simulink model "Both_Systems_GUI"  (R2020b)
settings: Solver=VariableStepAuto  StartTime=0.0  StopTime=10.0  RelTol=1e-3
model workspace (MAT data in the model file):
  Elev_Anti_friction = Simulink.Parameter
  Elev_Anti_friction.Value = 1
  Elev_Anti_friction.DataType = 'auto'
  Elev_Anti_friction.Dimensions = [1 1]
  Elev_Backlash = Simulink.Parameter
  Elev_Backlash.Value = 1
  Elev_Backlash.DataType = 'auto'
  Elev_Backlash.Dimensions = [1 1]
  Elev_CL = Simulink.Parameter
  Elev_CL.Value = 1
  Elev_CL.DataType = 'auto'
  Elev_CL.Dimensions = [1 1]
  Elev_Dist = Simulink.Parameter
  Elev_Dist.Value = 0
  Elev_Dist.DataType = 'auto'
  Elev_Dist.Dimensions = [1 1]
  Elev_Gun_Step = Simulink.Parameter
  Elev_Gun_Step.Value = 0
  Elev_Gun_Step.DataType = 'auto'
  Elev_Gun_Step.Dimensions = [1 1]
  Elev_Gun_Step_1_or_0_05 = Simulink.Parameter
  Elev_Gun_Step_1_or_0_05.Value = 1
  Elev_Gun_Step_1_or_0_05.DataType = 'auto'
  Elev_Gun_Step_1_or_0_05.Dimensions = [1 1]
  Elev_Input = Simulink.Parameter
  Elev_Input.Value = 1
  Elev_Input.DataType = 'auto'
  Elev_Input.Dimensions = [1 1]
  Elev_Insert_Input = Simulink.Parameter
  Elev_Insert_Input.Value = 0
  Elev_Insert_Input.DataType = 'auto'
  Elev_Insert_Input.Dimensions = [1 1]
  Elev_Optics_Enabled = Simulink.Parameter
  Elev_Optics_Enabled.Value = 1
  Elev_Optics_Enabled.DataType = 'auto'
  Elev_Optics_Enabled.Dimensions = [1 1]
  Elev_Pod_Backlash = Simulink.Parameter
  Elev_Pod_Backlash.Value = 1
  Elev_Pod_Backlash.DataType = 'auto'
  Elev_Pod_Backlash.Dimensions = [1 1]
  Elev_Pod_CL = Simulink.Parameter
  Elev_Pod_CL.Value = 1
  Elev_Pod_CL.DataType = 'auto'
  Elev_Pod_CL.Dimensions = [1 1]
  Elev_Pod_Friction = Simulink.Parameter
  Elev_Pod_Friction.Value = 1
  Elev_Pod_Friction.DataType = 'auto'
  Elev_Pod_Friction.Dimensions = [1 1]
  Elev_Pod_Step = Simulink.Parameter
  Elev_Pod_Step.Value = 0
  Elev_Pod_Step.DataType = 'auto'
  Elev_Pod_Step.Dimensions = [1 1]
  Elev_Pod_Step_1_or_0_05 = Simulink.Parameter
  Elev_Pod_Step_1_or_0_05.Value = 1
  Elev_Pod_Step_1_or_0_05.DataType = 'auto'
  Elev_Pod_Step_1_or_0_05.Dimensions = [1 1]
  Elev_Pod_Tacho = Simulink.Parameter
  Elev_Pod_Tacho.Value = 0
  Elev_Pod_Tacho.DataType = 'auto'
  Elev_Pod_Tacho.Dimensions = [1 1]
  Elev_Pod_hold = Simulink.Parameter
  Elev_Pod_hold.Value = 1
  Elev_Pod_hold.DataType = 'auto'
  Elev_Pod_hold.Dimensions = [1 1]
  Elev_Step_1_or_0_05 = Simulink.Parameter
  Elev_Step_1_or_0_05.Value = 1
  Elev_Step_1_or_0_05.DataType = 'auto'
  Elev_Step_1_or_0_05.Dimensions = [1 1]
  Elev_Tacho = Simulink.Parameter
  Elev_Tacho.Value = 0
  Elev_Tacho.DataType = 'auto'
  Elev_Tacho.Dimensions = [1 1]
  Elev_diffrentiator = Simulink.Parameter
  Elev_diffrentiator.Value = 1
  Elev_diffrentiator.DataType = 'auto'
  Elev_diffrentiator.Dimensions = [1 1]
  Elev_fire = Simulink.Parameter
  Elev_fire.Value = 1
  Elev_fire.DataType = 'auto'
  Elev_fire.Dimensions = [1 1]
  Elev_friction = Simulink.Parameter
  Elev_friction.Value = 1
  Elev_friction.DataType = 'auto'
  Elev_friction.Dimensions = [1 1]
  Trav_Anti_friction = Simulink.Parameter
  Trav_Anti_friction.Value = 1
  Trav_Anti_friction.DataType = 'auto'
  Trav_Anti_friction.Dimensions = [1 1]
  Trav_Backlash = Simulink.Parameter
  Trav_Backlash.Value = 1
  Trav_Backlash.DataType = 'auto'
  Trav_Backlash.Dimensions = [1 1]
  Trav_CL = Simulink.Parameter
  Trav_CL.Value = 1
  Trav_CL.DataType = 'auto'
  Trav_CL.Dimensions = [1 1]
  Trav_Dist = Simulink.Parameter
  Trav_Dist.Value = 1
  Trav_Dist.DataType = 'auto'
  Trav_Dist.Dimensions = [1 1]
  Trav_Gun_Step = Simulink.Parameter
  Trav_Gun_Step.Value = 0
  Trav_Gun_Step.DataType = 'auto'
  Trav_Gun_Step.Dimensions = [1 1]
  Trav_Gun_Step_1_or_0_05 = Simulink.Parameter
  Trav_Gun_Step_1_or_0_05.Value = 1
  Trav_Gun_Step_1_or_0_05.DataType = 'auto'
  Trav_Gun_Step_1_or_0_05.Dimensions = [1 1]
  Trav_Input = Simulink.Parameter
  Trav_Input.Value = 1
  Trav_Input.DataType = 'auto'
  Trav_Input.Dimensions = [1 1]
  Trav_Insert_Input = Simulink.Parameter
  Trav_Insert_Input.Value = 1
  Trav_Insert_Input.DataType = 'auto'
  Trav_Insert_Input.Dimensions = [1 1]
  Trav_Optics_Enabled = Simulink.Parameter
  Trav_Optics_Enabled.Value = 1
  Trav_Optics_Enabled.DataType = 'auto'
  Trav_Optics_Enabled.Dimensions = [1 1]
  Trav_Pod_Backlash = Simulink.Parameter
  Trav_Pod_Backlash.Value = 1
  Trav_Pod_Backlash.DataType = 'auto'
  Trav_Pod_Backlash.Dimensions = [1 1]
  Trav_Pod_CL = Simulink.Parameter
  Trav_Pod_CL.Value = 1
  Trav_Pod_CL.DataType = 'auto'
  Trav_Pod_CL.Dimensions = [1 1]
  Trav_Pod_Friction = Simulink.Parameter
  Trav_Pod_Friction.Value = 1
  Trav_Pod_Friction.DataType = 'auto'
  Trav_Pod_Friction.Dimensions = [1 1]
  Trav_Pod_Step = Simulink.Parameter
  Trav_Pod_Step.Value = 0
  Trav_Pod_Step.DataType = 'auto'
  Trav_Pod_Step.Dimensions = [1 1]
  Trav_Pod_Step_1_or_0_05 = Simulink.Parameter
  Trav_Pod_Step_1_or_0_05.Value = 1
  Trav_Pod_Step_1_or_0_05.DataType = 'auto'
  Trav_Pod_Step_1_or_0_05.Dimensions = [1 1]
  Trav_Pod_Tacho = Simulink.Parameter
  Trav_Pod_Tacho.Value = 0
  Trav_Pod_Tacho.DataType = 'auto'
  Trav_Pod_Tacho.Dimensions = [1 1]
  Trav_Pod_hold = Simulink.Parameter
  Trav_Pod_hold.Value = 1
  Trav_Pod_hold.DataType = 'auto'
  Trav_Pod_hold.Dimensions = [1 1]
  Trav_Step_1_or_0_05 = Simulink.Parameter
  Trav_Step_1_or_0_05.Value = 1
  Trav_Step_1_or_0_05.DataType = 'auto'
  Trav_Step_1_or_0_05.Dimensions = [1 1]
  Trav_Tacho = Simulink.Parameter
  Trav_Tacho.Value = 0
  Trav_Tacho.DataType = 'auto'
  Trav_Tacho.Dimensions = [1 1]
  Trav_diffrentiator = Simulink.Parameter
  Trav_diffrentiator.Value = 1
  Trav_diffrentiator.DataType = 'auto'
  Trav_diffrentiator.Dimensions = [1 1]
  Trav_fire = Simulink.Parameter
  Trav_fire.Value = 1
  Trav_fire.DataType = 'auto'
  Trav_fire.Dimensions = [1 1]
  Trav_friction = Simulink.Parameter
  Trav_friction.Value = 1
  Trav_friction.DataType = 'auto'
  Trav_friction.Dimensions = [1 1]
libraries: simulink x1
settings Model: Creator=דניאל ואיתי  LastModifiedBy=דניאל ואיתי

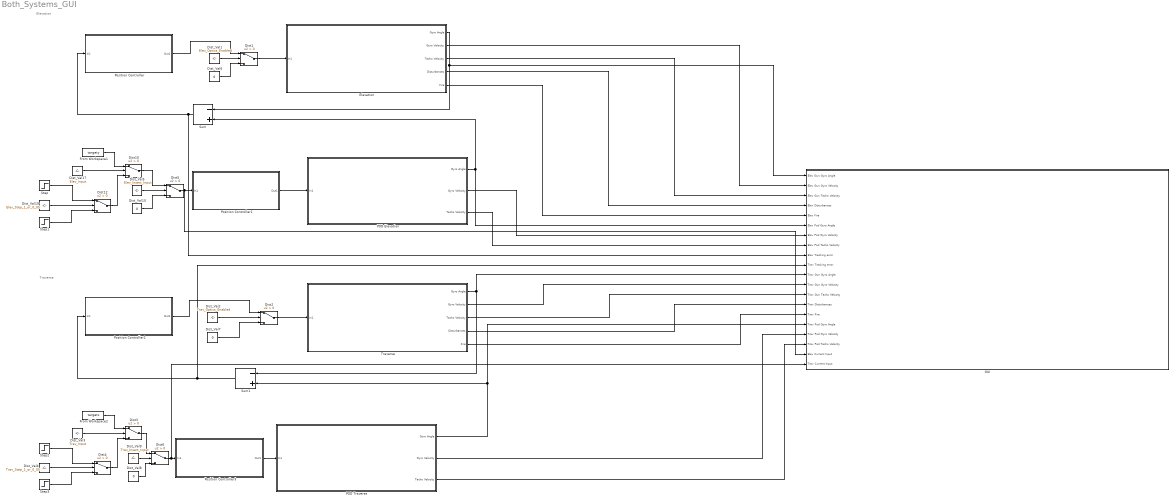
== system Both_Systems_GUI ==
  note: Elevation
  note: Traverse
  Dist{1..6,10,12} (8 alike) : Switch  Criteria=u2 > Threshold
  Dist_Val1 : Constant  Value=Elev_Optics_Enabled
  Dist_Val{6..8,10} (4 alike) : Constant  Value=0
  Dist_Val17 : Constant  Value=Elev_Input
  Dist_Val19 : Constant  Value=Elev_Step_1_or_0_05  VectorParams1D=off
  Dist_Val2 : Constant  Value=Trav_Optics_Enabled
  Dist_Val3 : Constant  Value=Trav_Input
  Dist_Val4 : Constant  Value=Trav_Step_1_or_0_05  VectorParams1D=off
  Dist_Val5 : Constant  Value=Elev_Insert_Input
  Dist_Val9 : Constant  Value=Trav_Insert_Input
  Elevation : Subsystem
  From Workspace1 : FromWorkspace  VariableName=targety
  From Workspace2 : FromWorkspace  VariableName=targetx
  GUI : Subsystem
  POD Elevation : Subsystem
  POD Traverse : Subsystem
  Position Controller : Subsystem
  Position Controller1 : Subsystem
  Position Controller2 : Subsystem
  Position Controller3 : Subsystem
  Step : Step  SampleTime=0
  Step1 : Step  After=0.05  SampleTime=0
  Step2 : Step  SampleTime=0
  Step3 : Step  After=0.05  SampleTime=0
  Sum : Sum  Inputs=-+
  Sum1 : Sum  Inputs=-+
  Traverse : Subsystem
  wires:
  Position Controller1/1(Out1) -> POD Elevation/1(In1)
  POD Elevation/2(Gyro Velocity) -> GUI/7(Elev Pod Gyro Velocity)
  Dist_Val17/1 -> Dist10/2
  From Workspace1/1 -> Dist10/1
  Step1/1 -> Dist12/3
  Elevation/3(Tacho Velocity) -> GUI/3(Elev Gun Tacho Velocity)
  POD Elevation/3(Tacho Velocity) -> GUI/8(Elev Pod Tacho Velocity)
  Elevation/2(Gyro Velocity) -> GUI/2(Elev Gun Gyro Velocity)
  Dist_Val1/1 -> Dist1/2
  Elevation/4(Disturbances) -> GUI/4(Elev Disturbances)
  POD Elevation/1(Gyro Angle) -> Sum/2, GUI/6(Elev Pod Gyro Angle)
  Step/1 -> Dist12/1
  Dist_Val19/1 -> Dist12/2
  Elevation/5(Fire) -> GUI/5(Elev Fire)
  Dist1/1 -> Elevation/1(In1)
  Dist12/1 -> Dist10/3
  Position Controller/1(Out1) -> Dist1/1
  Elevation/1(Gyro Angle) -> GUI/1(Elev Gun Gyro Angle), Sum/1
  Position Controller3/1(Out1) -> POD Traverse/1(In1)
  Dist2/1 -> Traverse/1(In1)
  Step2/1 -> Dist4/1
  Sum1/1 -> Position Controller2/1(In1), GUI/10(Trav Tracking error)
  From Workspace2/1 -> Dist3/1
  Dist4/1 -> Dist3/3
  Position Controller2/1(Out1) -> Dist2/1
  Step3/1 -> Dist4/3
  Dist_Val4/1 -> Dist4/2
  POD Traverse/1(Gyro Angle) -> GUI/16(Trav Pod Gyro Angle), Sum1/2
  Traverse/1(Gyro Angle) -> GUI/11(Trav Gun Gyro Angle), Sum1/1
  Dist_Val3/1 -> Dist3/2
  Dist_Val2/1 -> Dist2/2
  Traverse/2(Gyro Velocity) -> GUI/12(Trav Gun Gyro Velocity)
  Traverse/3(Tacho Velocity) -> GUI/13(Trav Gun Tacho Velocity)
  Traverse/4(Disturbances) -> GUI/14(Trav Disturbances)
  Traverse/5(Fire) -> GUI/15(Trav Fire)
  POD Traverse/2(Gyro Velocity) -> GUI/17(Trav Pod Gyro Velocity)
  POD Traverse/3(Tacho Velocity) -> GUI/18(Trav Pod Tacho Velocity)
  Dist5/1 -> GUI/19(Elev Current Input), Position Controller1/1(In1)
  Dist10/1 -> Dist5/1
  Dist_Val5/1 -> Dist5/2
  Dist_Val10/1 -> Dist5/3
  Dist_Val6/1 -> Dist1/3
  Dist_Val7/1 -> Dist2/3
  Dist6/1 -> GUI/20(Trav Current Input), Position Controller3/1(In1)
  Dist3/1 -> Dist6/1
  Dist_Val9/1 -> Dist6/2
  Dist_Val8/1 -> Dist6/3
  Sum/1 -> Position Controller/1(In1), GUI/9(Elev Tracking error)

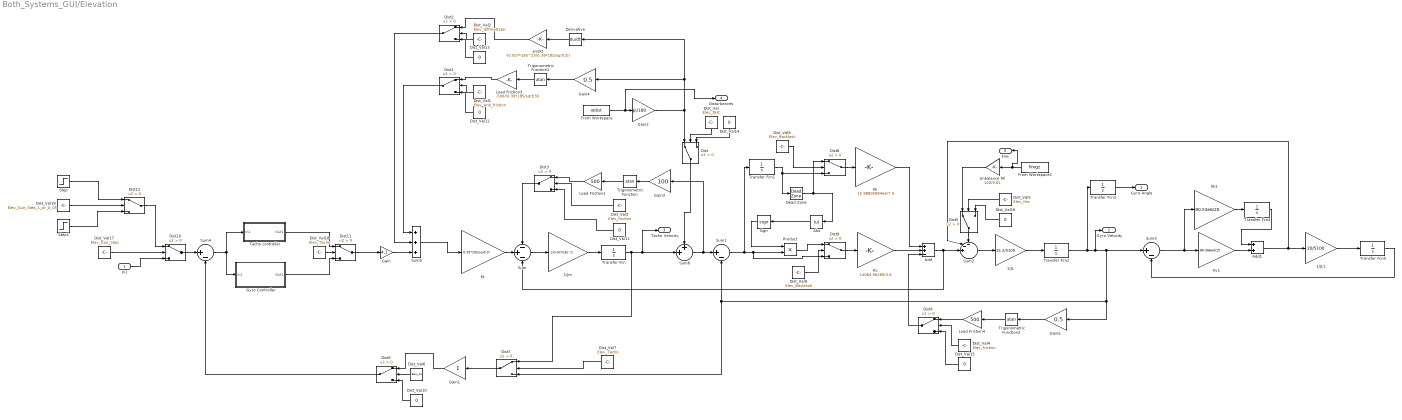
== system Both_Systems_GUI/Elevation ==
  In1 : Inport
  -Jm/Kt : Gain  Gain=-(0.007*185^2)/(0.39*185/sqrt(3))
  1/JL : Gain  Gain=15.2/5100
  1/JL1 : Gain  Gain=20/5100
  1/Jm : Gain  Gain=1/(0.007*185^2)
  Abs : Abs
  Add : Sum  Inputs=++-
  Add1 : Sum
  Dead Zone : DeadZone  LowerValue=-0.11e-3  UpperValue=0.11e-3  SaturateOnIntegerOverflow=on
  Derivative : Derivative
  Dist{,1..12} (13 alike) : Switch  Criteria=u2 > Threshold
  Dist_Val : Constant  Value=Elev_Dist
  Dist_Val1 : Constant  Value=Elev_Anti_friction
  Dist_Val{10..16} (7 alike) : Constant  Value=0
  Dist_Val17 : Constant  Value=Elev_Gun_Step
  Dist_Val18 : Constant  Value=Elev_Tacho
  Dist_Val19 : Constant  Value=Elev_Gun_Step_1_or_0_05
  Dist_Val2 : Constant  Value=Elev_diffrentiator
  Dist_Val3 : Constant  Value=Elev_friction
  Dist_Val4 : Constant  Value=Elev_friction
  Dist_Val5 : Constant  Value=Elev_fire
  Dist_Val6 : Constant  Value=Elev_CL
  Dist_Val7 : Constant  Value=Elev_Tacho
  Dist_Val8 : Constant  Value=Elev_Backlash
  Dist_Val9 : Constant  Value=Elev_Backlash
  From Workspace : FromWorkspace  VariableName=eldist  OutputAfterFinalValue=Setting to zero
  From Workspace1 : FromWorkspace  VariableName=firegz  OutputAfterFinalValue=Setting to zero
  Gain : Gain  Gain=4.1
  Gain1 : Gain
  Gain2 : Gain  Gain=pi/180
  Gain3 : Gain  Gain=100
  Gain4 : Gain  Gain=0.5
  Gain5 : Gain  Gain=0.5
  Gyro Controller : Subsystem
  Kk : Gain  Gain=15.98805984e6/7.9
  Kk1 : Gain  Gain=80.53e6/20
  Kt : Gain  Gain=0.39*185/sqrt(3)
  Kv : Gain  Gain=14084.96289/3.6
  Kv1 : Gain  Gain=80.366e3/15
  Load Friction1 : Gain  Gain=500
  Load Friction3 : Gain  Gain=-500/(0.39*185/sqrt(3))
  Load Friction4 : Gain  Gain=500
  Product : Product
  Sign : Signum
  Step : Step  SampleTime=0
  Step1 : Step  After=0.05  SampleTime=0
  Sum : Sum  Inputs=-+-
  Sum1 : Sum  Inputs=|+-
  Sum2 : Sum  Inputs=--+||
  Sum3 : Sum  Inputs=|+-
  Sum4 : Sum  Inputs=|+-
  Sum5 : Sum  Inputs=+++
  Sum8 : Sum  Inputs=++|
  Tacho controller : Subsystem
  Transfer Fcn{,1..5} (6 alike) : TransferFcn  Denominator=[1 0]
  Trigonometric Function : Trigonometry  Operator=atan
  Trigonometric Function1 : Trigonometry  Operator=atan
  Trigonometric Function2 : Trigonometry  Operator=atan
  Unbalance Ml : Gain  Gain=100/9.81
  Gyro Angle : Outport
  Gyro Velocity : Outport  Port=2
  Tacho Velocity : Outport  Port=3
  Disturbances : Outport  Port=4
  Fire : Outport  Port=5
  wires:
  Add/1 -> Sum/3, Sum2/3
  Kv/1 -> Add/2
  1/JL/1 -> Transfer Fcn2/1
  Sum/1 -> 1/Jm/1
  Kk/1 -> Add/1
  Kk1/1 -> Transfer Fcn4/1
  1/JL1/1 -> Transfer Fcn5/1
  Sum3/1 -> Kk1/1, Kv1/1
  Transfer Fcn4/1 -> Add1/1
  Kv1/1 -> Add1/2
  Transfer Fcn5/1 -> Sum3/2
  Sum2/1 -> 1/JL/1
  Add1/1 -> Sum2/2, 1/JL1/1
  Transfer Fcn2/1 -> Gyro Velocity/1, Sum1/2, Dist7/3, Gain5/1, Sum3/1, Transfer Fcn3/1
  Dist7/1 -> Gain1/1
  Sum4/1 -> Tacho controller/1(In1), Gyro Controller/1(In1)
  Tacho controller/1(Out1) -> Dist11/1
  Gyro Controller/1(Out1) -> Dist11/3
  Gain3/1 -> Trigonometric Function/1
  Trigonometric Function/1 -> Load Friction1/1
  Kt/1 -> Sum/2
  Trigonometric Function1/1 -> Load Friction3/1
  Sum5/1 -> Kt/1
  Gain5/1 -> Trigonometric Function2/1
  Trigonometric Function2/1 -> Load Friction4/1
  Transfer Fcn1/1 -> Dist8/3, Dead Zone/1
  Derivative/1 -> -Jm/Kt/1
  From Workspace1/1 -> Fire/1, Unbalance Ml/1
  1/Jm/1 -> Transfer Fcn/1
  Gain4/1 -> Trigonometric Function1/1
  Transfer Fcn/1 -> Dist7/1, Sum8/2, Tacho Velocity/1
  Dist11/1 -> Gain/1
  Gain/1 -> Sum5/3
  Sum1/1 -> Dist9/3, Product/2, Transfer Fcn1/1
  Abs/1 -> Sign/1
  Sign/1 -> Product/1
  From Workspace/1 -> Disturbances/1, Gain2/1
  Sum8/1 -> Sum1/1, Gain3/1
  Step/1 -> Dist12/1
  Dist_Val19/1 -> Dist12/2
  Step1/1 -> Dist12/3
  Dist12/1 -> Dist10/1
  In1/1 -> Dist10/3
  Dist_Val17/1 -> Dist10/2
  Dist10/1 -> Sum4/1
  Dist_Val18/1 -> Dist11/2
  Dist_Val6/1 -> Dist6/2
  Dist_Val10/1 -> Dist6/3
  Gain1/1 -> Dist6/1
  Dist_Val7/1 -> Dist7/2
  Dist_Val11/1 -> Dist3/3
  Dist_Val3/1 -> Dist3/2
  Load Friction1/1 -> Dist3/1
  Dist3/1 -> Sum/1
  -Jm/Kt/1 -> Dist2/1
  Load Friction3/1 -> Dist1/1
  Dist_Val1/1 -> Dist1/2
  Dist_Val2/1 -> Dist2/2
  Dist_Val13/1 -> Dist2/3
  Dist_Val12/1 -> Dist1/3
  Dist1/1 -> Sum5/1
  Dist2/1 -> Sum5/2
  Dist_Val14/1 -> Dist/3
  Dist_Val/1 -> Dist/2
  Gain2/1 -> Derivative/1, Gain4/1, Dist/1
  Dist/1 -> Sum8/1
  Dist_Val8/1 -> Dist8/2
  Dist8/1 -> Kk/1
  Dead Zone/1 -> Abs/1, Dist8/1
  Dist_Val9/1 -> Dist9/2
  Dist9/1 -> Kv/1
  Product/1 -> Dist9/1
  Dist_Val5/1 -> Dist5/2
  Dist_Val16/1 -> Dist5/3
  Dist5/1 -> Sum2/1
  Unbalance Ml/1 -> Dist5/1
  Dist_Val4/1 -> Dist4/2
  Dist_Val15/1 -> Dist4/3
  Load Friction4/1 -> Dist4/1
  Dist4/1 -> Add/3
  Transfer Fcn3/1 -> Gyro Angle/1
  Dist6/1 -> Sum4/2

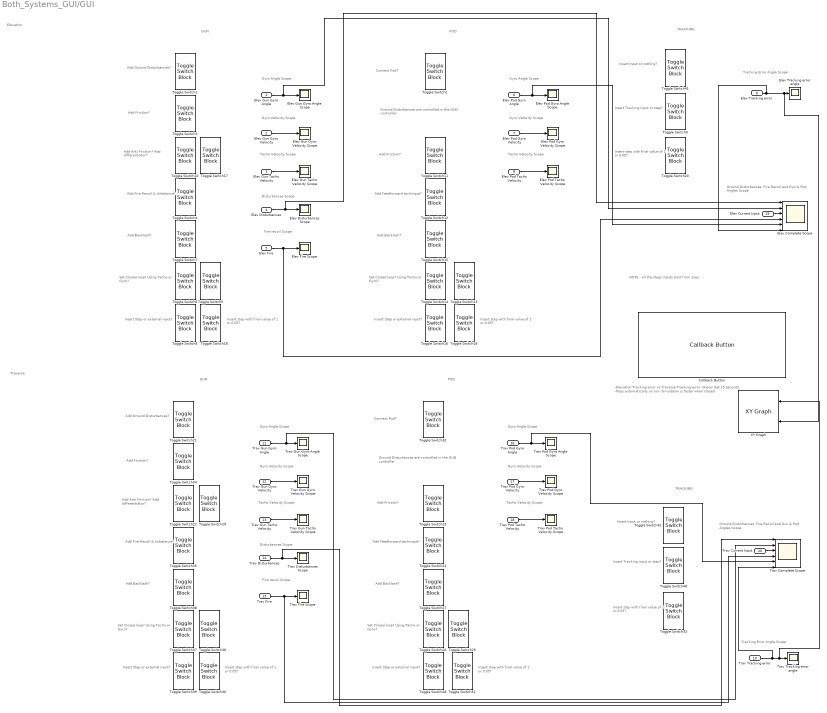
== system Both_Systems_GUI/GUI ==
  note: Add Ground
      | Disturbances?
  note: GUN
  note: Add Friction?
  note: Add Fire Recoil
      | & Unbalance?
  note: Add Backlash?
  note: Set Closed loop?
      | Using Tacho or Gyro?
  note: Insert Step
      | or external input?
  note: Gyro Angle Scope
  note: Gyro Velocity Scope
  note: Tacho Velocity Scope
  note: Disturbances Scope
  note: Fire recoil Scope
  note: Add Friction?
  note: Add Feedforward
      | technique?
  note: Ground Disturbances are
      | controlled in the GUN controller
  note: Gyro Angle Scope
  note: Gyro Velocity Scope
  note: Tacho Velocity Scope
  note: Insert Step
      | or external input?
  note: Add Backlash?
  note: Set Closed loop?
      | Using Tacho or Gyro?
  note: POD
  note: TRACKING
  note: Tracking Error Angle Scope
  note: Insert Tracking
      | input or step?
  note: Add Anti Friction?
      | Add differentiator?
  note: Connect Pod?
  note: Insert step with final
      | value of 1 or 0.05?
  note: Insert step with final
      | value of 1 or 0.05?
  note: Insert step with final
      | value of 1 or 0.05?
  note: NOTE - all the steps inputs start from 1sec
  note: TRACKING
  note: Tracking Error Angle Scope
  note: Insert Tracking
      | input or step?
  note: Insert step with final
      | value of 1 or 0.05?
  note: Elevation
  note: Traverse
  note: Set Closed loop?
      | Using Tacho or Gyro?
  note: Fire recoil Scope
  note: Disturbances Scope
  note: Tacho Velocity Scope
  note: Add Friction?
  note: Add Fire Recoil
      | & Unbalance?
  note: Insert Step
      | or external input?
  note: Gyro Angle Scope
  note: Gyro Velocity Scope
  note: Add Backlash?
  note: Insert Step
      | or external input?
  note: Add Friction?
  note: Ground Disturbances are
      | controlled in the GUN controller
  note: Add Ground
      | Disturbances?
  note: Add Backlash?
  note: Gyro Angle Scope
  note: GUN
  note: Gyro Velocity Scope
  note: Tacho Velocity Scope
  note: Insert step with final
      | value of 1 or 0.05?
  note: Insert step with final
      | value of 1 or 0.05?
  note: Add Feedforward
      | technique?
  note: Connect Pod?
  note: Add Anti Friction?
      | Add differentiator?
  note: POD
  note: Set Closed loop?
      | Using Tacho or Gyro?
  note: -Elevation Tracking error vs Traverse Tracking error
      | -Shows last 15 seconds
      | -Pops automatically on run
      | -Simulation is faster when closed
  note: Insert Input
      | or nothing?
  note: Insert Input
      | or nothing?
  note: Ground Disturbances, Fire Recoil
      | and Gun & Pod Angles Scope
  note: Ground Disturbances, Fire Recoil
      | and Gun & Pod Angles Scope
  Elev Gun Gyro Angle : Inport
  Elev Gun Gyro Velocity : Inport  Port=2
  Elev Gun Tacho Velocity : Inport  Port=3
  Elev Disturbances : Inport  Port=4
  Elev Fire : Inport  Port=5
  Elev Pod Gyro Angle : Inport  Port=6
  Elev Pod Gyro Velocity : Inport  Port=7
  Elev Pod Tacho Velocity : Inport  Port=8
  Elev Tracking error : Inport  Port=9
  Trav Tracking error : Inport  Port=10
  Trav Gun Gyro Angle : Inport  Port=11
  Trav Gun Gyro Velocity : Inport  Port=12
  Trav Gun Tacho Velocity : Inport  Port=13
  Trav Disturbances : Inport  Port=14
  Trav Fire : Inport  Port=15
  Trav Pod Gyro Angle : Inport  Port=16
  Trav Pod Gyro Velocity : Inport  Port=17
  Trav Pod Tacho Velocity : Inport  Port=18
  Elev Current Input : Inport  Port=19
  Trav Current Input : Inport  Port=20
  Callback Button : CallbackButton  ButtonText=RUN
      settings: ClickFcn=|
      | mdlWks = get_param('Both_Systems_GUI','ModelWorkspace');
      | dist = getVariable(mdlWks, "Trav_Dist");
      | fire = getVariable(mdlWks, "Trav_fire");
      | track = getVariable(mdlWks, "Trav_Input");
      | trackInsert = getVariable(mdlWks, "Trav_Insert_Input");
      | dist2 = getVariable(mdlWks, "Elev_Dist");
      | fire2 = getVariable(mdlWks, "Elev_fire");
      | track2 = getVariable(mdlWks, "Elev_Input");
      | trackInsert2 = getVariable(mdlWks, "Elev_Insert_Input");
      | 
      | if((track.Value == 1 && trackInsert.Value == 1) || (track2.Value == 1 && trackInsert2.Value == 1))
      |     sim(bdroot, [0 45]);
      | elseif (dist.Value == 1 || dist2.Value == 1)
      |     sim(bdroot, [0 20]);
      | elseif (fire.Value == 1 || fire2.Value == 1)
      |     sim(bdroot, [0 16]);
      | else
      |     sim(bdroot, [0 10]);
      | end
  Elev Complete Scope : Scope  NumInputPorts=6
  Elev Disturbances Scope : Scope
  Elev Fire Scope : Scope
  Elev Gun Gyro Angle Scope : Scope
  Elev Gun Gyro Velocity Scope : Scope
  Elev Gun Tacho Velocity Scope : Scope
  Elev Pod Gyro Angle Scope : Scope
  Elev Pod Gyro Velocity Scope : Scope
  Elev Pod Tacho Velocity Scope : Scope
  Elev Tracking error angle : Scope
  Toggle Switch{1..42} (42 alike) : ToggleSwitchBlock
      settings: Values={{'Off', 'On'}, [0 1]}
  Trav Complete Scope : Scope  NumInputPorts=6
  Trav Disturbances Scope : Scope
  Trav Fire Scope : Scope
  Trav Gun Gyro Angle Scope : Scope
  Trav Gun Gyro Velocity Scope : Scope
  Trav Gun Tacho Velocity Scope : Scope
  Trav Pod Gyro Angle Scope : Scope
  Trav Pod Gyro Velocity Scope : Scope
  Trav Pod Tacho Velocity Scope : Scope
  Trav Tracking error angle : Scope
  XY Graph : simulink/Sinks/XY Graph  xmin=-5e-4  xmax=5e-4  ymin=-8e-4  ymax=8e-4  st=-1
  wires:
  Elev Gun Gyro Angle/1 -> Elev Complete Scope/2, Elev Gun Gyro Angle Scope/1
  Elev Gun Gyro Velocity/1 -> Elev Gun Gyro Velocity Scope/1
  Elev Disturbances/1 -> Elev Complete Scope/1, Elev Disturbances Scope/1
  Elev Fire/1 -> Elev Complete Scope/4, Elev Fire Scope/1
  Elev Gun Tacho Velocity/1 -> Elev Gun Tacho Velocity Scope/1
  Elev Pod Gyro Velocity/1 -> Elev Pod Gyro Velocity Scope/1
  Elev Pod Tacho Velocity/1 -> Elev Pod Tacho Velocity Scope/1
  Elev Pod Gyro Angle/1 -> Elev Complete Scope/5, Elev Pod Gyro Angle Scope/1
  Elev Tracking error/1 -> Elev Complete Scope/6, XY Graph/2, Elev Tracking error angle/1
  Trav Tracking error/1 -> Trav Complete Scope/6, XY Graph/1, Trav Tracking error angle/1
  Trav Pod Gyro Velocity/1 -> Trav Pod Gyro Velocity Scope/1
  Trav Pod Gyro Angle/1 -> Trav Complete Scope/5, Trav Pod Gyro Angle Scope/1
  Trav Pod Tacho Velocity/1 -> Trav Pod Tacho Velocity Scope/1
  Trav Gun Tacho Velocity/1 -> Trav Gun Tacho Velocity Scope/1
  Trav Gun Gyro Velocity/1 -> Trav Gun Gyro Velocity Scope/1
  Trav Fire/1 -> Trav Complete Scope/4, Trav Fire Scope/1
  Trav Gun Gyro Angle/1 -> Trav Complete Scope/2, Trav Gun Gyro Angle Scope/1
  Trav Disturbances/1 -> Trav Complete Scope/1, Trav Disturbances Scope/1
  Trav Current Input/1 -> Trav Complete Scope/3
  Elev Current Input/1 -> Elev Complete Scope/3

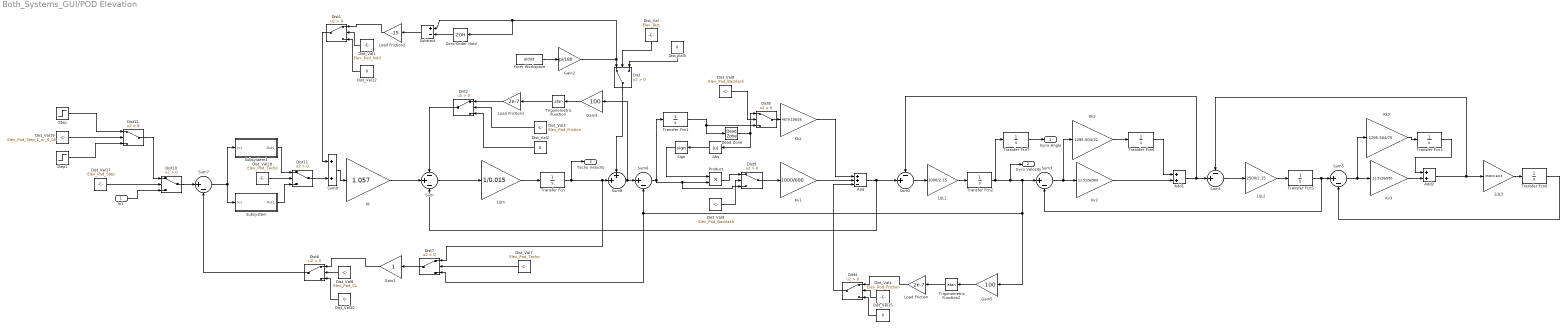
== system Both_Systems_GUI/POD Elevation ==
  In1 : Inport
  1/JL1 : Gain  Gain=1000/2.15
  1/JL2 : Gain  Gain=2500/2.15
  1/JL3 : Gain  Gain=2500/0.6215
  1/Jm : Gain  Gain=1/0.015
  Abs : Abs
  Add : Sum  Inputs=++-
  Add1 : Sum
  Add2 : Sum
  Dead Zone : DeadZone  LowerValue=-0.07e-5  UpperValue=0.07e-5  SaturateOnIntegerOverflow=on
  Dist{,1..2,4,6..12} (11 alike) : Switch  Criteria=u2 > Threshold
  Dist_Val : Constant  Value=Elev_Dist
  Dist_Val1 : Constant  Value=Elev_Pod_hold
  Dist_Val{2,5,10,12,15} (5 alike) : Constant  Value=0
  Dist_Val17 : Constant  Value=Elev_Pod_Step
  Dist_Val18 : Constant  Value=Elev_Pod_Tacho
  Dist_Val19 : Constant  Value=Elev_Pod_Step_1_or_0_05
  Dist_Val3 : Constant  Value=Elev_Pod_Friction
  Dist_Val4 : Constant  Value=Elev_Pod_Friction
  Dist_Val6 : Constant  Value=Elev_Pod_CL
  Dist_Val7 : Constant  Value=Elev_Pod_Tacho
  Dist_Val8 : Constant  Value=Elev_Pod_Backlash
  Dist_Val9 : Constant  Value=Elev_Pod_Backlash
  From Workspace : FromWorkspace  VariableName=eldist  OutputAfterFinalValue=Setting to zero
  Gain1 : Gain
  Gain2 : Gain  Gain=pi/180
  Gain3 : Gain  Gain=100
  Gain5 : Gain  Gain=100
  Kk1 : Gain  Gain=4679.199/26
  Kk2 : Gain  Gain=1295.504/32
  Kk3 : Gain  Gain=1295.504/75
  Kt : Gain  Gain=1.057
  Kv1 : Gain  Gain=1000/600
  Kv2 : Gain  Gain=11.5126/500
  Kv3 : Gain  Gain=11.5126/650
  Load Friction : Gain  Gain=2e-7
  Load Friction1 : Gain  Gain=2e-7
  Load Friction2 : Gain  Gain=-15
  Product : Product
  Sign : Signum
  Step : Step  SampleTime=0
  Step1 : Step  After=0.05  SampleTime=0
  Subsystem : Subsystem
  Subsystem1 : Subsystem
  Subtract : Sum  Inputs=+-
  Sum : Sum  Inputs=-+-
  Sum1 : Sum  Inputs=-+|
  Sum2 : Sum  Inputs=-+|
  Sum{3,5..7} (4 alike) : Sum  Inputs=|+-
  Sum8 : Sum  Inputs=++|
  Sum9 : Sum
  Transfer Fcn{,1..7} (8 alike) : TransferFcn  Denominator=[1 0]
  Trigonometric Function : Trigonometry  Operator=atan
  Trigonometric Function2 : Trigonometry  Operator=atan
  Zero-Order Hold : ZeroOrderHold  SampleTime=0.001
  Gyro Angle : Outport
  Gyro Velocity : Outport  Port=2
  Tacho Velocity : Outport  Port=3
  wires:
  Kk1/1 -> Add/1
  Kt/1 -> Sum/2
  Sum/1 -> 1/Jm/1
  Kv1/1 -> Add/2
  1/Jm/1 -> Transfer Fcn/1
  Sum2/1 -> 1/JL1/1
  1/JL1/1 -> Transfer Fcn2/1
  Add/1 -> Sum2/2, Sum/3
  Transfer Fcn5/1 -> Sum3/2, Sum5/1
  Transfer Fcn4/1 -> Add1/1
  Kk2/1 -> Transfer Fcn4/1
  1/JL2/1 -> Transfer Fcn5/1
  Sum3/1 -> Kk2/1, Kv2/1
  Kv2/1 -> Add1/2
  Add1/1 -> Sum1/2, Sum2/1
  Sum7/1 -> Subsystem1/1(In1), Subsystem/1(In1)
  Sum1/1 -> 1/JL2/1
  Add2/1 -> 1/JL3/1, Sum1/1
  1/JL3/1 -> Transfer Fcn6/1
  Kk3/1 -> Transfer Fcn3/1
  Sum5/1 -> Kk3/1, Kv3/1
  Transfer Fcn3/1 -> Add2/1
  Kv3/1 -> Add2/2
  Transfer Fcn6/1 -> Sum5/2
  Transfer Fcn2/1 -> Gyro Velocity/1, Dist7/3, Sum6/2, Gain5/1, Sum3/1, Transfer Fcn7/1
  Transfer Fcn/1 -> Dist7/1, Sum8/2, Tacho Velocity/1
  Sum8/1 -> Gain3/1, Sum6/1
  Subsystem1/1(Out1) -> Dist11/1
  Sum9/1 -> Kt/1
  Dist11/1 -> Sum9/2
  Gain2/1 -> Dist/1, Subtract/1, Zero-Order Hold/1
  Gain3/1 -> Trigonometric Function/1
  Trigonometric Function/1 -> Load Friction1/1
  Abs/1 -> Sign/1
  Sum6/1 -> Dist9/3, Product/2, Transfer Fcn1/1
  Dead Zone/1 -> Dist8/1, Abs/1
  Transfer Fcn1/1 -> Dead Zone/1, Dist8/3
  Sign/1 -> Product/1
  Trigonometric Function2/1 -> Load Friction/1
  Gain5/1 -> Trigonometric Function2/1
  Transfer Fcn7/1 -> Gyro Angle/1
  From Workspace/1 -> Gain2/1
  Zero-Order Hold/1 -> Subtract/2
  Subtract/1 -> Load Friction2/1
  Dist_Val15/1 -> Dist4/3
  Load Friction/1 -> Dist4/1
  Dist_Val4/1 -> Dist4/2
  Dist4/1 -> Add/3
  Dist_Val8/1 -> Dist8/2
  Dist8/1 -> Kk1/1
  Dist_Val9/1 -> Dist9/2
  Product/1 -> Dist9/1
  Dist9/1 -> Kv1/1
  Dist_Val6/1 -> Dist6/2
  Dist_Val10/1 -> Dist6/3
  Gain1/1 -> Dist6/1
  Dist6/1 -> Sum7/2
  Dist_Val7/1 -> Dist7/2
  Dist7/1 -> Gain1/1
  Step1/1 -> Dist12/3
  Step/1 -> Dist12/1
  Dist_Val19/1 -> Dist12/2
  In1/1 -> Dist10/3
  Dist_Val17/1 -> Dist10/2
  Dist12/1 -> Dist10/1
  Dist_Val18/1 -> Dist11/2
  Subsystem/1(Out1) -> Dist11/3
  Dist_Val2/1 -> Dist2/3
  Dist_Val3/1 -> Dist2/2
  Load Friction1/1 -> Dist2/1
  Dist2/1 -> Sum/1
  Load Friction2/1 -> Dist1/1
  Dist_Val1/1 -> Dist1/2
  Dist_Val12/1 -> Dist1/3
  Dist1/1 -> Sum9/1
  Dist_Val5/1 -> Dist/3
  Dist_Val/1 -> Dist/2
  Dist/1 -> Sum8/1
  Dist10/1 -> Sum7/1

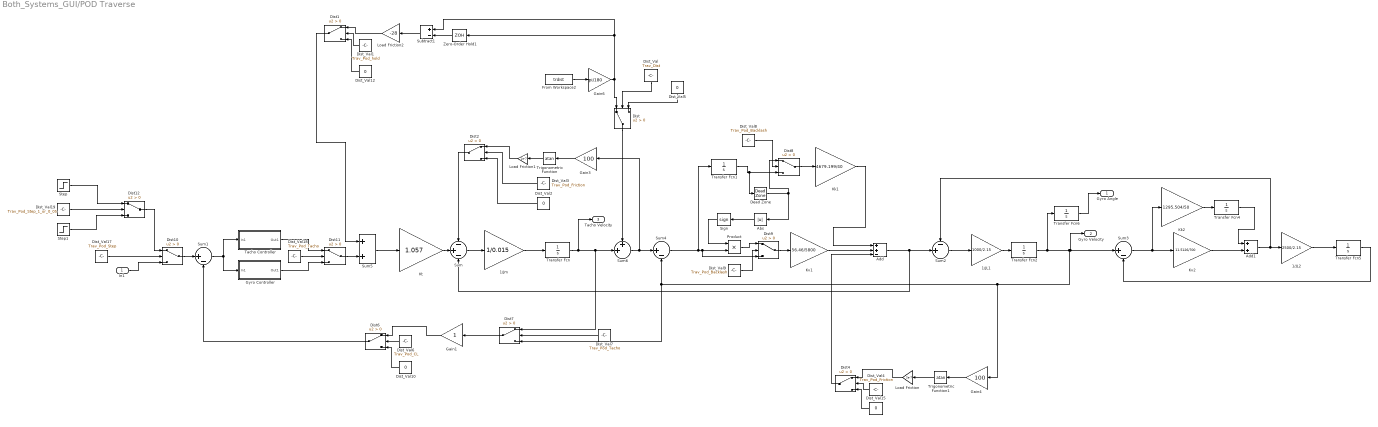
== system Both_Systems_GUI/POD Traverse ==
  In1 : Inport
  1/JL1 : Gain  Gain=1000/2.15
  1/JL2 : Gain  Gain=2500/2.15
  1/Jm : Gain  Gain=1/0.015
  Abs : Abs
  Add : Sum  Inputs=++-
  Add1 : Sum
  Dead Zone : DeadZone  LowerValue=-0.07e-5  UpperValue=0.07e-5  SaturateOnIntegerOverflow=on
  Dist{,1..2,4,6..12} (11 alike) : Switch  Criteria=u2 > Threshold
  Dist_Val : Constant  Value=Trav_Dist
  Dist_Val1 : Constant  Value=Trav_Pod_hold
  Dist_Val{2,5,10,12,15} (5 alike) : Constant  Value=0
  Dist_Val17 : Constant  Value=Trav_Pod_Step
  Dist_Val18 : Constant  Value=Trav_Pod_Tacho
  Dist_Val19 : Constant  Value=Trav_Pod_Step_1_or_0_05
  Dist_Val3 : Constant  Value=Trav_Pod_Friction
  Dist_Val4 : Constant  Value=Trav_Pod_Friction
  Dist_Val6 : Constant  Value=Trav_Pod_CL
  Dist_Val7 : Constant  Value=Trav_Pod_Tacho
  Dist_Val8 : Constant  Value=Trav_Pod_Backlash
  Dist_Val9 : Constant  Value=Trav_Pod_Backlash
  From Workspace2 : FromWorkspace  VariableName=trdist  OutputAfterFinalValue=Setting to zero
  Gain1 : Gain
  Gain3 : Gain  Gain=100
  Gain4 : Gain  Gain=100
  Gain6 : Gain  Gain=pi/180
  Gyro Controller : Subsystem
  Kk1 : Gain  Gain=4679.199/40
  Kk2 : Gain  Gain=1295.504/50
  Kt : Gain  Gain=1.057
  Kv1 : Gain  Gain=56.46/5800
  Kv2 : Gain  Gain=11.5126/700
  Load Friction : Gain  Gain=2e-7
  Load Friction1 : Gain  Gain=2e-7
  Load Friction2 : Gain  Gain=-28
  Product : Product
  Sign : Signum
  Step : Step  SampleTime=0
  Step1 : Step  After=0.05  SampleTime=0
  Subtract1 : Sum  Inputs=+-
  Sum : Sum  Inputs=-+-
  Sum1 : Sum  Inputs=|+-
  Sum2 : Sum  Inputs=-+|
  Sum3 : Sum  Inputs=|+-
  Sum4 : Sum  Inputs=|+-
  Sum5 : Sum
  Sum6 : Sum  Inputs=++|
  Tacho Controller : Subsystem
  Transfer Fcn{,1..2,4..6} (6 alike) : TransferFcn  Denominator=[1 0]
  Trigonometric Function : Trigonometry  Operator=atan
  Trigonometric Function1 : Trigonometry  Operator=atan
  Zero-Order Hold1 : ZeroOrderHold  SampleTime=0.001
  Gyro Angle : Outport
  Gyro Velocity : Outport  Port=2
  Tacho Velocity : Outport  Port=3
  wires:
  Kk1/1 -> Add/1
  Kt/1 -> Sum/2
  Sum/1 -> 1/Jm/1
  Kv1/1 -> Add/2
  1/Jm/1 -> Transfer Fcn/1
  Sum2/1 -> 1/JL1/1
  1/JL1/1 -> Transfer Fcn2/1
  Add/1 -> Sum/3, Sum2/2
  Transfer Fcn5/1 -> Sum3/2
  Transfer Fcn4/1 -> Add1/1
  Kk2/1 -> Transfer Fcn4/1
  Sum3/1 -> Kv2/1, Kk2/1
  Kv2/1 -> Add1/2
  Add1/1 -> 1/JL2/1, Sum2/1
  1/JL2/1 -> Transfer Fcn5/1
  Transfer Fcn/1 -> Dist7/1, Sum6/2, Tacho Velocity/1
  Dist7/1 -> Gain1/1
  Sum1/1 -> Tacho Controller/1(In1), Gyro Controller/1(In1)
  From Workspace2/1 -> Gain6/1
  Sum4/1 -> Product/2, Dist9/3, Transfer Fcn1/1
  Trigonometric Function/1 -> Load Friction1/1
  Gain3/1 -> Trigonometric Function/1
  Sum6/1 -> Gain3/1, Sum4/1
  Dead Zone/1 -> Dist8/1, Abs/1
  Transfer Fcn1/1 -> Dist8/3, Dead Zone/1
  Abs/1 -> Sign/1
  Sign/1 -> Product/1
  Trigonometric Function1/1 -> Load Friction/1
  Gain4/1 -> Trigonometric Function1/1
  Transfer Fcn2/1 -> Dist7/3, Sum4/2, Gain4/1, Sum3/1, Gyro Velocity/1, Transfer Fcn6/1
  Transfer Fcn6/1 -> Gyro Angle/1
  Gain6/1 -> Dist/1, Zero-Order Hold1/1, Subtract1/1
  Subtract1/1 -> Load Friction2/1
  Zero-Order Hold1/1 -> Subtract1/2
  Dist10/1 -> Sum1/1
  Dist_Val/1 -> Dist/2
  Dist_Val4/1 -> Dist4/2
  Dist_Val15/1 -> Dist4/3
  Load Friction/1 -> Dist4/1
  Dist8/1 -> Kk1/1
  Dist_Val8/1 -> Dist8/2
  Product/1 -> Dist9/1
  Dist9/1 -> Kv1/1
  Dist_Val9/1 -> Dist9/2
  Load Friction2/1 -> Dist1/1
  Dist_Val1/1 -> Dist1/2
  Dist_Val12/1 -> Dist1/3
  Dist_Val2/1 -> Dist2/3
  Dist_Val3/1 -> Dist2/2
  Load Friction1/1 -> Dist2/1
  Dist_Val5/1 -> Dist/3
  Dist_Val10/1 -> Dist6/3
  Dist_Val6/1 -> Dist6/2
  Gain1/1 -> Dist6/1
  Dist_Val7/1 -> Dist7/2
  In1/1 -> Dist10/3
  Dist_Val17/1 -> Dist10/2
  Dist_Val18/1 -> Dist11/2
  Tacho Controller/1(Out1) -> Dist11/1
  Gyro Controller/1(Out1) -> Dist11/3
  Step/1 -> Dist12/1
  Dist_Val19/1 -> Dist12/2
  Step1/1 -> Dist12/3
  Dist12/1 -> Dist10/1
  Sum5/1 -> Kt/1
  Dist11/1 -> Sum5/2
  Dist1/1 -> Sum5/1
  Dist2/1 -> Sum/1
  Dist/1 -> Sum6/1
  Dist6/1 -> Sum1/2
  Dist4/1 -> Add/3

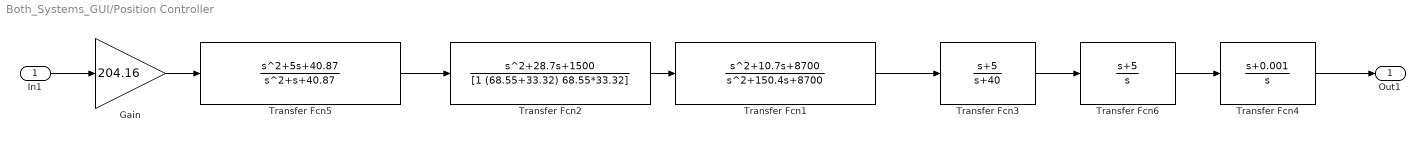
== system Both_Systems_GUI/Position Controller ==
  In1 : Inport
  Gain : Gain  Gain=204.16
  Transfer Fcn1 : TransferFcn  Numerator=[1 10.7 8700]  Denominator=[1 150.4 8700]
  Transfer Fcn2 : TransferFcn  Numerator=[1 28.7 1500]  Denominator=[1 (68.55+33.32) 68.55*33.32]
  Transfer Fcn3 : TransferFcn  Numerator=[1 5]  Denominator=[1 40]
  Transfer Fcn4 : TransferFcn  Numerator=[1 0.001]  Denominator=[1 0]
  Transfer Fcn5 : TransferFcn  Numerator=[1 5 40.87]  Denominator=[1 1 40.87]
  Transfer Fcn6 : TransferFcn  Numerator=[1 5]  Denominator=[1 0]
  Out1 : Outport
  wires:
  Transfer Fcn1/1 -> Transfer Fcn3/1
  Transfer Fcn2/1 -> Transfer Fcn1/1
  Transfer Fcn5/1 -> Transfer Fcn2/1
  Gain/1 -> Transfer Fcn5/1
  Transfer Fcn3/1 -> Transfer Fcn6/1
  In1/1 -> Gain/1
  Transfer Fcn6/1 -> Transfer Fcn4/1
  Transfer Fcn4/1 -> Out1/1

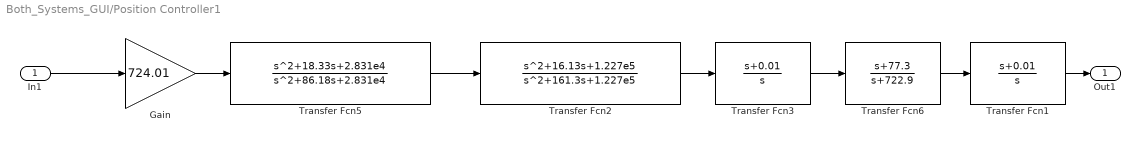
== system Both_Systems_GUI/Position Controller1 ==
  In1 : Inport
  Gain : Gain  Gain=724.01
  Transfer Fcn1 : TransferFcn  Numerator=[1 0.01]  Denominator=[1 0]
  Transfer Fcn2 : TransferFcn  Numerator=[1 16.13 1.227e5]  Denominator=[1 161.3 1.227e5]
  Transfer Fcn3 : TransferFcn  Numerator=[1 0.01]  Denominator=[1 0]
  Transfer Fcn5 : TransferFcn  Numerator=[1 18.33 2.831e4]  Denominator=[1 86.18 2.831e4]
  Transfer Fcn6 : TransferFcn  Numerator=[1 77.3]  Denominator=[1 722.9]
  Out1 : Outport
  wires:
  In1/1 -> Gain/1
  Transfer Fcn2/1 -> Transfer Fcn3/1
  Transfer Fcn5/1 -> Transfer Fcn2/1
  Gain/1 -> Transfer Fcn5/1
  Transfer Fcn3/1 -> Transfer Fcn6/1
  Transfer Fcn1/1 -> Out1/1
  Transfer Fcn6/1 -> Transfer Fcn1/1

== system Both_Systems_GUI/Position Controller2 ==
  In1 : Inport
  Gain : Gain  Gain=782.55
  Transfer Fcn : TransferFcn  Numerator=[1 2]  Denominator=[1 0]
  Transfer Fcn1 : TransferFcn  Numerator=[1 10]  Denominator=[1 0]
  Transfer Fcn2 : TransferFcn  Numerator=[1 35.05 675.6]  Denominator=[1 (15.32+754.8) 15.32*754.8]
  Transfer Fcn3 : TransferFcn  Numerator=[1 22.58 4.12e4]  Denominator=[1 49 4.12e4]
  Out1 : Outport
  wires:
  Gain/1 -> Transfer Fcn/1
  In1/1 -> Gain/1
  Transfer Fcn/1 -> Transfer Fcn2/1
  Transfer Fcn2/1 -> Transfer Fcn3/1
  Transfer Fcn1/1 -> Out1/1
  Transfer Fcn3/1 -> Transfer Fcn1/1

== system Both_Systems_GUI/Position Controller3 ==
  In1 : Inport
  Gain : Gain  Gain=2573.5
  Transfer Fcn1 : TransferFcn  Numerator=[1 0.001]  Denominator=[1 0]
  Transfer Fcn3 : TransferFcn  Numerator=[1 0.001]  Denominator=[1 0]
  Transfer Fcn5 : TransferFcn  Numerator=[1 76.22 2.501e4]  Denominator=[1 (253.4*2) 253.4^2]
  Transfer Fcn6 : TransferFcn  Numerator=[1 49.39]  Denominator=[1 786.1]
  Out1 : Outport
  wires:
  In1/1 -> Gain/1
  Transfer Fcn5/1 -> Transfer Fcn3/1
  Gain/1 -> Transfer Fcn5/1
  Transfer Fcn3/1 -> Transfer Fcn6/1
  Transfer Fcn1/1 -> Out1/1
  Transfer Fcn6/1 -> Transfer Fcn1/1

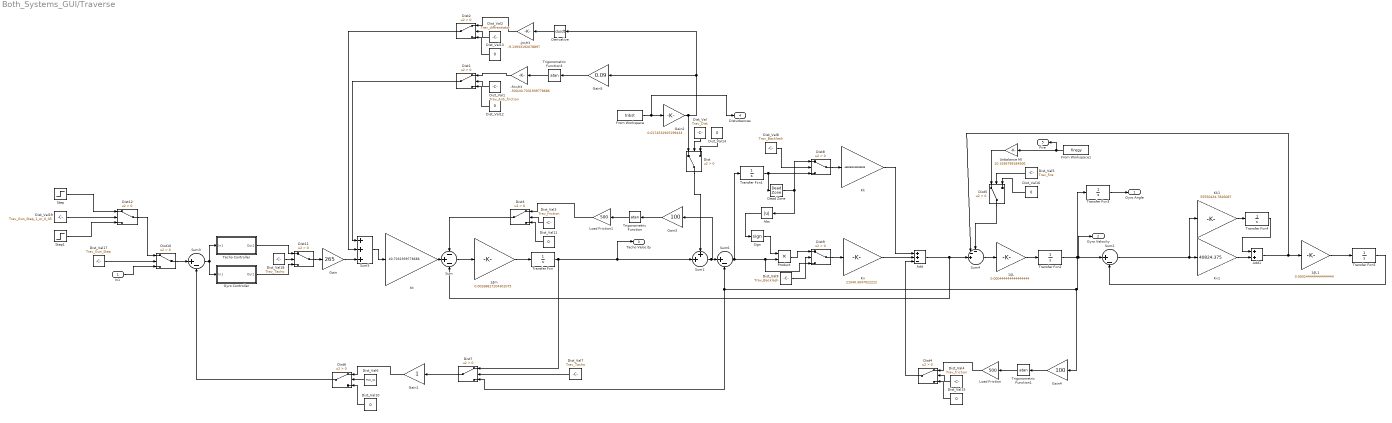
== system Both_Systems_GUI/Traverse ==
  In1 : Inport
  -Jm/Kt : Gain  Gain=-9.13933192078897
  -fric/Kt : Gain  Gain=-500/40.7031939778686
  1/JL : Gain  Gain=0.000444444444444444
  1/JL1 : Gain  Gain=0.000244444444444444
  1/Jm : Gain  Gain=0.00268817204301075
  Abs : Abs
  Add : Sum  Inputs=++-
  Add1 : Sum
  Dead Zone : DeadZone  LowerValue=-0.11e-3  UpperValue=0.11e-3  SaturateOnIntegerOverflow=on
  Derivative : Derivative
  Dist{,1..12} (13 alike) : Switch  Criteria=u2 > Threshold
  Dist_Val : Constant  Value=Trav_Dist
  Dist_Val1 : Constant  Value=Trav_Anti_friction
  Dist_Val{10..16} (7 alike) : Constant  Value=0
  Dist_Val17 : Constant  Value=Trav_Gun_Step
  Dist_Val18 : Constant  Value=Trav_Tacho
  Dist_Val19 : Constant  Value=Trav_Gun_Step_1_or_0_05
  Dist_Val2 : Constant  Value=Trav_diffrentiator
  Dist_Val3 : Constant  Value=Trav_friction
  Dist_Val4 : Constant  Value=Trav_friction
  Dist_Val5 : Constant  Value=Trav_fire
  Dist_Val6 : Constant  Value=Trav_CL
  Dist_Val7 : Constant  Value=Trav_Tacho
  Dist_Val8 : Constant  Value=Trav_Backlash
  Dist_Val9 : Constant  Value=Trav_Backlash
  From Workspace : FromWorkspace  VariableName=trdist  OutputAfterFinalValue=Setting to zero
  From Workspace1 : FromWorkspace  VariableName=firegy  OutputAfterFinalValue=Setting to zero
  Gain : Gain  Gain=265
  Gain1 : Gain
  Gain2 : Gain  Gain=0.0174532925199433
  Gain3 : Gain  Gain=100
  Gain4 : Gain  Gain=100
  Gain5 : Gain  Gain=0.09
  Gyro Controller : Subsystem
  Kk : Gain  Gain=4692605.90333333
  Kk1 : Gain  Gain=55550434.7826087
  Kt : Gain  Gain=40.7031939778686
  Kv : Gain  Gain=21040.3047022222
  Kv1 : Gain  Gain=40824.375
  Load Friction : Gain  Gain=500
  Load Friction1 : Gain  Gain=500
  Product : Product
  Sign : Signum
  Step : Step  SampleTime=0
  Step1 : Step  After=0.05  SampleTime=0
  Sum : Sum  Inputs=-+-
  Sum1 : Sum  Inputs=++|
  Sum2 : Sum  Inputs=|+-
  Sum3 : Sum  Inputs=|+-
  Sum4 : Sum  Inputs=--+||
  Sum5 : Sum  Inputs=+++
  Sum6 : Sum  Inputs=|+-
  Tacho Controller : Subsystem
  Transfer Fcn{,1..5} (6 alike) : TransferFcn  Numerator=1  Denominator=[1 0]
  Trigonometric Function : Trigonometry  Operator=atan
  Trigonometric Function1 : Trigonometry  Operator=atan
  Trigonometric Function3 : Trigonometry  Operator=atan
  Unbalance Ml : Gain  Gain=10.1936799184506
  Gyro Angle : Outport
  Gyro Velocity : Outport  Port=2
  Tacho Velocity : Outport  Port=3
  Disturbances : Outport  Port=4
  Fire : Outport  Port=5
  wires:
  Add/1 -> Sum4/3, Sum/3
  Kv/1 -> Add/2
  1/JL/1 -> Transfer Fcn2/1
  1/Jm/1 -> Transfer Fcn/1
  Sum/1 -> 1/Jm/1
  Kk/1 -> Add/1
  Sum5/1 -> Kt/1
  Kk1/1 -> Transfer Fcn4/1
  Add1/1 -> Sum4/2, 1/JL1/1
  Sum2/1 -> Kk1/1, Kv1/1
  Transfer Fcn5/1 -> Sum2/2
  Kv1/1 -> Add1/2
  Transfer Fcn4/1 -> Add1/1
  1/JL1/1 -> Transfer Fcn5/1
  Sum4/1 -> 1/JL/1
  Sum3/1 -> Gyro Controller/1(In1), Tacho Controller/1(In1)
  Dist7/1 -> Gain1/1
  From Workspace/1 -> Disturbances/1, Gain2/1
  Transfer Fcn2/1 -> Transfer Fcn3/1, Gyro Velocity/1, Sum2/1, Sum6/2, Dist7/3, Gain4/1
  Dist11/1 -> Gain/1
  Gain/1 -> Sum5/3
  Trigonometric Function1/1 -> Load Friction/1
  Derivative/1 -> -Jm/Kt/1
  Trigonometric Function/1 -> Load Friction1/1
  Transfer Fcn3/1 -> Gyro Angle/1
  Gain3/1 -> Trigonometric Function/1
  Gain4/1 -> Trigonometric Function1/1
  From Workspace1/1 -> Unbalance Ml/1, Fire/1
  Trigonometric Function3/1 -> -fric/Kt/1
  Gain5/1 -> Trigonometric Function3/1
  Transfer Fcn/1 -> Dist7/1, Tacho Velocity/1, Sum1/2
  Kt/1 -> Sum/2
  Dead Zone/1 -> Abs/1, Dist8/1
  Sign/1 -> Product/1
  Abs/1 -> Sign/1
  Sum6/1 -> Dist9/3, Product/2, Transfer Fcn1/1
  Sum1/1 -> Gain3/1, Sum6/1
  Transfer Fcn1/1 -> Dist8/3, Dead Zone/1
  Dist10/1 -> Sum3/1
  Gain2/1 -> Derivative/1, Gain5/1, Dist/1
  Unbalance Ml/1 -> Dist5/1
  Dist/1 -> Sum1/1
  Dist_Val/1 -> Dist/2
  Dist_Val1/1 -> Dist1/2
  -fric/Kt/1 -> Dist1/1
  Dist1/1 -> Sum5/1
  Dist_Val2/1 -> Dist2/2
  -Jm/Kt/1 -> Dist2/1
  Dist2/1 -> Sum5/2
  Dist_Val3/1 -> Dist3/2
  Load Friction1/1 -> Dist3/1
  Dist3/1 -> Sum/1
  Load Friction/1 -> Dist4/1
  Dist_Val4/1 -> Dist4/2
  Dist4/1 -> Add/3
  Dist_Val5/1 -> Dist5/2
  Dist5/1 -> Sum4/1
  Gain1/1 -> Dist6/1
  Dist_Val6/1 -> Dist6/2
  Dist6/1 -> Sum3/2
  Dist_Val7/1 -> Dist7/2
  Dist_Val8/1 -> Dist8/2
  Dist8/1 -> Kk/1
  Dist9/1 -> Kv/1
  Dist_Val9/1 -> Dist9/2
  Product/1 -> Dist9/1
  Dist_Val10/1 -> Dist6/3
  Dist_Val11/1 -> Dist3/3
  Dist_Val12/1 -> Dist1/3
  Dist_Val13/1 -> Dist2/3
  Dist_Val14/1 -> Dist/3
  Dist_Val15/1 -> Dist4/3
  Dist_Val16/1 -> Dist5/3
  Dist_Val17/1 -> Dist10/2
  In1/1 -> Dist10/3
  Dist_Val18/1 -> Dist11/2
  Tacho Controller/1(Out1) -> Dist11/1
  Gyro Controller/1(Out1) -> Dist11/3
  Dist_Val19/1 -> Dist12/2
  Step/1 -> Dist12/1
  Step1/1 -> Dist12/3
  Dist12/1 -> Dist10/1

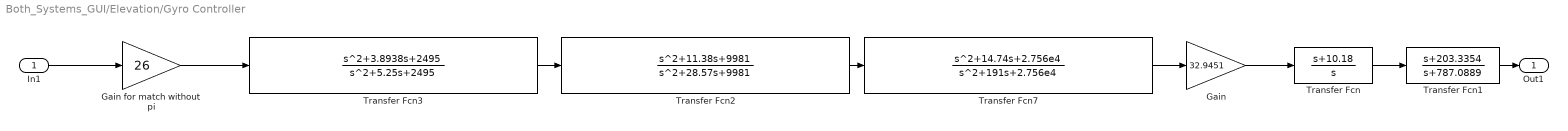
== system Both_Systems_GUI/Elevation/Gyro Controller ==
  In1 : Inport
  Gain : Gain  Gain=32.9451
  Gain for match without pi : Gain  Gain=26
  Transfer Fcn : TransferFcn  Numerator=[1 10.18]  Denominator=[1 0]
  Transfer Fcn1 : TransferFcn  Numerator=[1 203.3354]  Denominator=[1 787.0889]
  Transfer Fcn2 : TransferFcn  Numerator=[1 11.38 9981]  Denominator=[1 28.57 9981]
  Transfer Fcn3 : TransferFcn  Numerator=[1 3.8938 2495]  Denominator=[1 5.25 2495]
  Transfer Fcn7 : TransferFcn  Numerator=[1 14.74 2.756e4]  Denominator=[1 191 2.756e4]
  Out1 : Outport
  wires:
  Gain/1 -> Transfer Fcn/1
  Gain for match without pi/1 -> Transfer Fcn3/1
  In1/1 -> Gain for match without pi/1
  Transfer Fcn/1 -> Transfer Fcn1/1
  Transfer Fcn1/1 -> Out1/1
  Transfer Fcn2/1 -> Transfer Fcn7/1
  Transfer Fcn3/1 -> Transfer Fcn2/1
  Transfer Fcn7/1 -> Gain/1

== system Both_Systems_GUI/Elevation/Tacho controller ==
  In1 : Inport
  Transfer Fcn2 : TransferFcn  Numerator=[1 313.6]  Denominator=[1 35.33]
  Transfer Fcn4 : TransferFcn  Numerator=[1 20.77 1.017e4]  Denominator=[1 65.67 1.017e4]
  Transfer Fcn5 : TransferFcn  Numerator=[1 0.0001]  Denominator=[1 0]
  a5 : Gain  Gain=129.13
  Out1 : Outport
  wires:
  In1/1 -> Transfer Fcn4/1
  a5/1 -> Transfer Fcn5/1
  Transfer Fcn4/1 -> Transfer Fcn2/1
  Transfer Fcn5/1 -> Out1/1
  Transfer Fcn2/1 -> a5/1

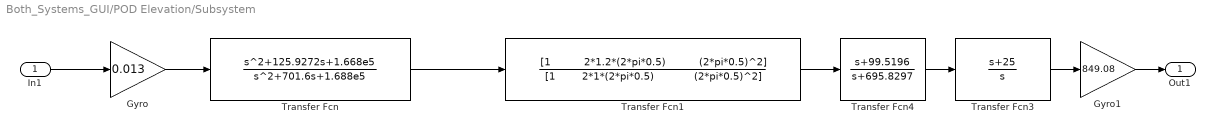
== system Both_Systems_GUI/POD Elevation/Subsystem ==
  In1 : Inport
  Gyro : Gain  Gain=0.013
  Gyro1 : Gain  Gain=849.08
  Transfer Fcn : TransferFcn  Numerator=[1 125.9272 1.668e5]  Denominator=[1 701.6 1.688e5]
  Transfer Fcn1 : TransferFcn  Numerator="[1          2*1.2*(2*pi*0.5)          (2*pi*0.5)^2]"  Denominator="[1        2*1*(2*pi*0.5)            (2*pi*0.5)^2]"
  Transfer Fcn3 : TransferFcn  Numerator=[1 25]  Denominator=[1 0]
  Transfer Fcn4 : TransferFcn  Numerator=[1 99.5196]  Denominator=[1 695.8297]
  Out1 : Outport
  wires:
  In1/1 -> Gyro/1
  Gyro1/1 -> Out1/1
  Gyro/1 -> Transfer Fcn/1
  Transfer Fcn4/1 -> Transfer Fcn3/1
  Transfer Fcn3/1 -> Gyro1/1
  Transfer Fcn/1 -> Transfer Fcn1/1
  Transfer Fcn1/1 -> Transfer Fcn4/1

== system Both_Systems_GUI/POD Elevation/Subsystem1 ==
  In1 : Inport
  Gyro : Gain  Gain=0.015
  Gyro1 : Gain  Gain=165.71
  Transfer Fcn1 : TransferFcn  Numerator=[1 91.51 4.836e4]  Denominator=[1 145 4.836e4]
  Transfer Fcn3 : TransferFcn  Numerator=[1 3.5]  Denominator=[1 0]
  Out1 : Outport
  wires:
  In1/1 -> Gyro/1
  Transfer Fcn1/1 -> Transfer Fcn3/1
  Gyro/1 -> Transfer Fcn1/1
  Transfer Fcn3/1 -> Gyro1/1
  Gyro1/1 -> Out1/1

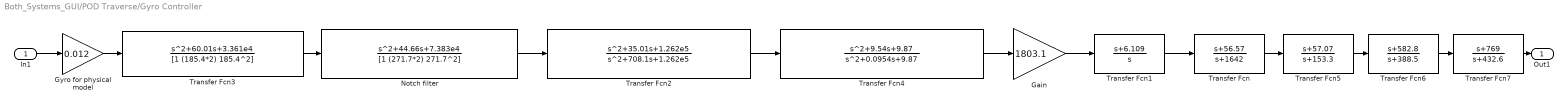
== system Both_Systems_GUI/POD Traverse/Gyro Controller ==
  In1 : Inport
  Gain : Gain  Gain=1803.1
  Gyro for physical model : Gain  Gain=0.012
  Notch filter : TransferFcn  Numerator=[1 44.66 7.383e4]  Denominator=[1 (271.7*2) 271.7^2]
  Transfer Fcn : TransferFcn  Numerator=[1 56.57]  Denominator=[1 1642]
  Transfer Fcn1 : TransferFcn  Numerator=[1 6.109]  Denominator=[1 0]
  Transfer Fcn2 : TransferFcn  Numerator=[1 35.01 1.262e5]  Denominator=[1 708.1 1.262e5]
  Transfer Fcn3 : TransferFcn  Numerator=[1 60.01 3.361e4]  Denominator=[1 (185.4*2) 185.4^2]
  Transfer Fcn4 : TransferFcn  Numerator=[1 9.54 9.87]  Denominator=[1 0.0954 9.87]
  Transfer Fcn5 : TransferFcn  Numerator=[1 57.07]  Denominator=[1 153.3]
  Transfer Fcn6 : TransferFcn  Numerator=[1 582.8]  Denominator=[1 388.5]
  Transfer Fcn7 : TransferFcn  Numerator=[1 769]  Denominator=[1 432.6]
  Out1 : Outport
  wires:
  Notch filter/1 -> Transfer Fcn2/1
  Gain/1 -> Transfer Fcn1/1
  Transfer Fcn1/1 -> Transfer Fcn/1
  In1/1 -> Gyro for physical model/1
  Transfer Fcn3/1 -> Notch filter/1
  Gyro for physical model/1 -> Transfer Fcn3/1
  Transfer Fcn2/1 -> Transfer Fcn4/1
  Transfer Fcn4/1 -> Gain/1
  Transfer Fcn5/1 -> Transfer Fcn6/1
  Transfer Fcn/1 -> Transfer Fcn5/1
  Transfer Fcn6/1 -> Transfer Fcn7/1
  Transfer Fcn7/1 -> Out1/1

== system Both_Systems_GUI/POD Traverse/Tacho Controller ==
  In1 : Inport
  Gain : Gain  Gain=76.091
  Gain for physical fit : Gain  Gain=0.017
  Transfer Fcn : TransferFcn  Numerator=[1 0.5]  Denominator=[1 0]
  Transfer Fcn1 : TransferFcn  Numerator=[1 52.43 2.419e4]  Denominator=[1 165.6 2.419e4]
  Transfer Fcn2 : TransferFcn  Numerator=[1 38.45 7.643e4]  Denominator=[1 384.5 7.643e4]
  Out1 : Outport
  wires:
  Gain/1 -> Transfer Fcn/1
  In1/1 -> Gain for physical fit/1
  Gain for physical fit/1 -> Gain/1
  Transfer Fcn/1 -> Transfer Fcn1/1
  Transfer Fcn1/1 -> Transfer Fcn2/1
  Transfer Fcn2/1 -> Out1/1

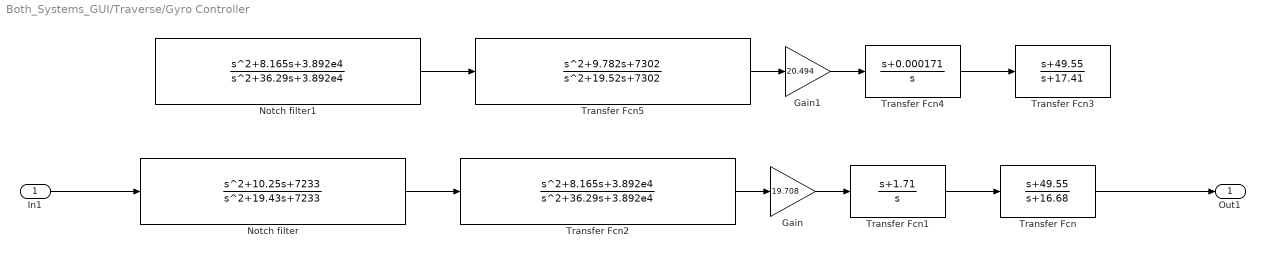
== system Both_Systems_GUI/Traverse/Gyro Controller ==
  In1 : Inport
  Gain : Gain  Gain=19.708
  Gain1 : Gain  Gain=20.494
  Notch filter : TransferFcn  Numerator=[1 10.25 7233]  Denominator=[1 19.43 7233]
  Notch filter1 : TransferFcn  Numerator=[1 8.165 3.892e4]  Denominator=[1 36.29 3.892e4]
  Transfer Fcn : TransferFcn  Numerator=[1 49.55]  Denominator=[1 16.68]
  Transfer Fcn1 : TransferFcn  Numerator=[1 1.71]  Denominator=[1 0]
  Transfer Fcn2 : TransferFcn  Numerator=[1 8.165 3.892e4]  Denominator=[1 36.29 3.892e4]
  Transfer Fcn3 : TransferFcn  Numerator=[1 49.55]  Denominator=[1 17.41]
  Transfer Fcn4 : TransferFcn  Numerator=[1 0.000171]  Denominator=[1 0]
  Transfer Fcn5 : TransferFcn  Numerator=[1 9.782 7302]  Denominator=[1 19.52 7302]
  Out1 : Outport
  wires:
  Notch filter/1 -> Transfer Fcn2/1
  Transfer Fcn2/1 -> Gain/1
  Gain/1 -> Transfer Fcn1/1
  Transfer Fcn1/1 -> Transfer Fcn/1
  Transfer Fcn4/1 -> Transfer Fcn3/1
  Gain1/1 -> Transfer Fcn4/1
  Transfer Fcn5/1 -> Gain1/1
  Notch filter1/1 -> Transfer Fcn5/1
  Transfer Fcn/1 -> Out1/1
  In1/1 -> Notch filter/1

== system Both_Systems_GUI/Traverse/Tacho Controller ==
  In1 : Inport
  Gain : Gain  Gain=28.117
  Transfer Fcn : TransferFcn  Numerator=[1 20.07 1.322e4]  Denominator=[1 80.27 1.322e4]
  Transfer Fcn1 : TransferFcn  Numerator=[1 2*0.1*2*pi*4.24 (2*pi*4.24)^2]  Denominator=[1 2*0.4*2*pi*4.24 (2*pi*4.24)^2]
  Transfer Fcn2 : TransferFcn  Numerator=[1 14.31]  Denominator=[1 31.36]
  Transfer Fcn3 : TransferFcn  Numerator=[1 359.4]  Denominator=[1 40.5]
  Transfer Fcn4 : TransferFcn  Numerator=[1 0.0001]  Denominator=[1 0]
  Out1 : Outport
  wires:
  In1/1 -> Transfer Fcn/1
  Gain/1 -> Transfer Fcn4/1
  Transfer Fcn4/1 -> Transfer Fcn2/1
  Transfer Fcn/1 -> Gain/1
  Transfer Fcn2/1 -> Transfer Fcn3/1
  Transfer Fcn3/1 -> Out1/1
